simulink model "FullDPDDesign"  (R2015a)
settings: Solver=ode45  SolverMode=SingleTasking  StartTime=0.0  StopTime=1000000  RelTol=1e-3
undefined symbols (not defined in the file): CC1, CC2, gcbh, xlBlockLoadCallback, xlGetNormalizedPeriod, xlipgetpartsetting
libraries: xbsIndex_r4 x211
(part 2 of 2)

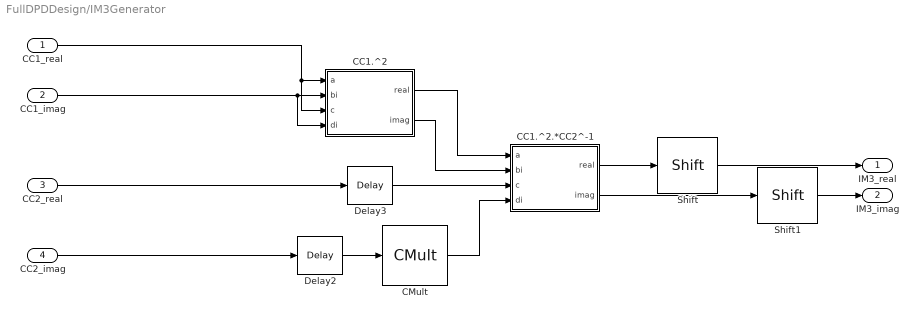
== system FullDPDDesign/IM3Generator ==
  CC1_real : Inport
  CC1_imag : Inport  Port=2
  CC2_real : Inport  Port=3
  CC2_imag : Inport  Port=4
  CC1.^2 : Subsystem
  CC1.^2.*CC2^-1 : Subsystem
  CMult : xbsIndex_r4/CMult  const=-1  gui_display_data_type=Fixed-point  const_n_bits=16  const_bin_pt=14  float_type=Single  exp_bits=8  fraction_bits=24  en=off  latency=0  precision=User Defined  arith_type="Signed  (2's comp)"  n_bits=16  bin_pt=14  quantization=Truncate  overflow=Wrap  dbl_ovrd=off  use_behavioral_HDL=off  mem_type=Distributed RAM  pipeline=off  block_type=cmult
  Delay2 : xbsIndex_r4/Delay  rst=off  infoeditControl=Selection of Reset will increase slice count due to use of real FFs and instead of SRLs  en=off  latency=4  dbl_ovrd=off  reg_retiming=off  block_type=delay
  Delay3 : xbsIndex_r4/Delay  rst=off  infoeditControl=Selection of Reset will increase slice count due to use of real FFs and instead of SRLs  en=off  latency=4  dbl_ovrd=off  reg_retiming=off  block_type=delay
  Shift : xbsIndex_r4/Shift  shift_dir=Left  shift_bits=2  en=off  latency=0  precision=Full  arith_type="Signed  (2's comp)"  n_bits=16  bin_pt=14  quantization=Truncate  overflow=Wrap  dbl_ovrd=off  block_type=shift
  Shift1 : xbsIndex_r4/Shift  shift_dir=Left  shift_bits=2  en=off  latency=0  precision=Full  arith_type="Signed  (2's comp)"  n_bits=16  bin_pt=14  quantization=Truncate  overflow=Wrap  dbl_ovrd=off  block_type=shift
  IM3_real : Outport
  IM3_imag : Outport  Port=2
  wires:
  CC1.^2/1(real) -> CC1.^2.*CC2^-1/1(a)
  Delay3/1 -> CC1.^2.*CC2^-1/3(c)
  CMult/1 -> CC1.^2.*CC2^-1/4(di)
  CC1.^2/2(imag) -> CC1.^2.*CC2^-1/2(bi)
  Delay2/1 -> CMult/1
  CC2_real/1 -> Delay3/1
  CC2_imag/1 -> Delay2/1
  CC1_real/1 -> CC1.^2/3(c), CC1.^2/1(a)
  CC1_imag/1 -> CC1.^2/2(bi), CC1.^2/4(di)
  CC1.^2.*CC2^-1/1(real) -> Shift/1
  CC1.^2.*CC2^-1/2(imag) -> Shift1/1
  Shift/1 -> IM3_real/1
  Shift1/1 -> IM3_imag/1

== system FullDPDDesign/IM3RotationGenerator ==
  Counter1 : xbsIndex_r4/Counter  cnt_type=Count Limited  cnt_to=39  operation=Up  start_count=0  cnt_by_val=1  arith_type=Unsigned  n_bits=6  bin_pt=0  load_pin=off  rst=off  en=off  explicit_period=on  period=1  dbl_ovrd=off  use_behavioral_HDL=off  implementation=Fabric  block_type=counter
  Negate1 : xbsIndex_r4/Negate  precision=User Defined  arith_type="Signed  (2's comp)"  n_bits=16  bin_pt=14  quantization=Truncate  overflow=Wrap  en=off  latency=0  dbl_ovrd=off  block_type=negate
  ROM : xbsIndex_r4/ROM  depth=40  initVector=cos(2*pi*(1:40)*9/40)  distributed_mem=Block RAM  rst=off  init_reg=0  en=off  latency=12  gui_display_data_type=Fixed-point  arith_type="Signed  (2's comp)"  n_bits=16  bin_pt=14  preci_type=Single  exp_width=8  frac_width=24  dbl_ovrd=off  optimize=Area  use_rpm=on  block_type=sprom
  ROM1 : xbsIndex_r4/ROM  depth=40  initVector=sin(2*pi*(1:40)*9/40)  distributed_mem=Block RAM  rst=off  init_reg=0  en=off  latency=12  gui_display_data_type=Fixed-point  arith_type="Signed  (2's comp)"  n_bits=16  bin_pt=14  preci_type=Single  exp_width=8  frac_width=24  dbl_ovrd=off  optimize=Area  use_rpm=on  block_type=sprom
  Rotate_real : Outport
  -Rotate_imag : Outport  Port=2
  Rotate_imag : Outport  Port=3
  wires:
  Counter1/1 -> ROM1/1, ROM/1
  ROM1/1 -> Negate1/1, Rotate_imag/1
  ROM/1 -> Rotate_real/1
  Negate1/1 -> -Rotate_imag/1

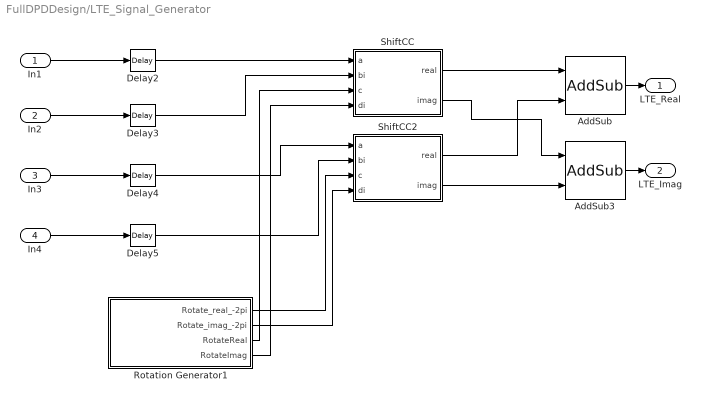
== system FullDPDDesign/LTE_Signal_Generator ==
  In1 : Inport
  In2 : Inport  Port=2
  In3 : Inport  Port=3
  In4 : Inport  Port=4
  AddSub : xbsIndex_r4/AddSub  mode=Addition  use_carryin=off  use_carryout=off  en=off  latency=3+8  precision=User Defined  arith_type="Signed  (2's comp)"  n_bits=16  bin_pt=14  quantization="Round  (unbiased: +/- Inf)"  overflow=Saturate  dbl_ovrd=off  use_behavioral_HDL=off  hw_selection=Fabric  pipelined=off  block_type=addsub
  AddSub3 : xbsIndex_r4/AddSub  mode=Addition  use_carryin=off  use_carryout=off  en=off  latency=3+8  precision=User Defined  arith_type="Signed  (2's comp)"  n_bits=16  bin_pt=14  quantization="Round  (unbiased: +/- Inf)"  overflow=Saturate  dbl_ovrd=off  use_behavioral_HDL=off  hw_selection=Fabric  pipelined=off  block_type=addsub
  Delay{2..5} (4 alike) : xbsIndex_r4/Delay  rst=off  infoeditControl=Selection of Reset will increase slice count due to use of real FFs and instead of SRLs  en=off  latency=1  dbl_ovrd=off  reg_retiming=off  block_type=delay
  Rotation Generator1 : Subsystem
  ShiftCC : Subsystem
  ShiftCC2 : Subsystem
  LTE_Real : Outport
  LTE_Imag : Outport  Port=2
  wires:
  In4/1 -> Delay5/1
  Delay3/1 -> ShiftCC/2(bi)
  Rotation Generator1/3(RotateReal) -> ShiftCC/3(c)
  Rotation Generator1/1(Rotate_real_-2pi) -> ShiftCC2/3(c)
  Delay5/1 -> ShiftCC2/2(bi)
  Delay4/1 -> ShiftCC2/1(a)
  Delay2/1 -> ShiftCC/1(a)
  Rotation Generator1/4(RotateImag) -> ShiftCC/4(di)
  In2/1 -> Delay3/1
  In3/1 -> Delay4/1
  Rotation Generator1/2(Rotate_imag_-2pi) -> ShiftCC2/4(di)
  ShiftCC/1(real) -> AddSub/1
  ShiftCC2/2(imag) -> AddSub3/2
  ShiftCC/2(imag) -> AddSub3/1
  ShiftCC2/1(real) -> AddSub/2
  AddSub3/1 -> LTE_Imag/1
  AddSub/1 -> LTE_Real/1
  In1/1 -> Delay2/1

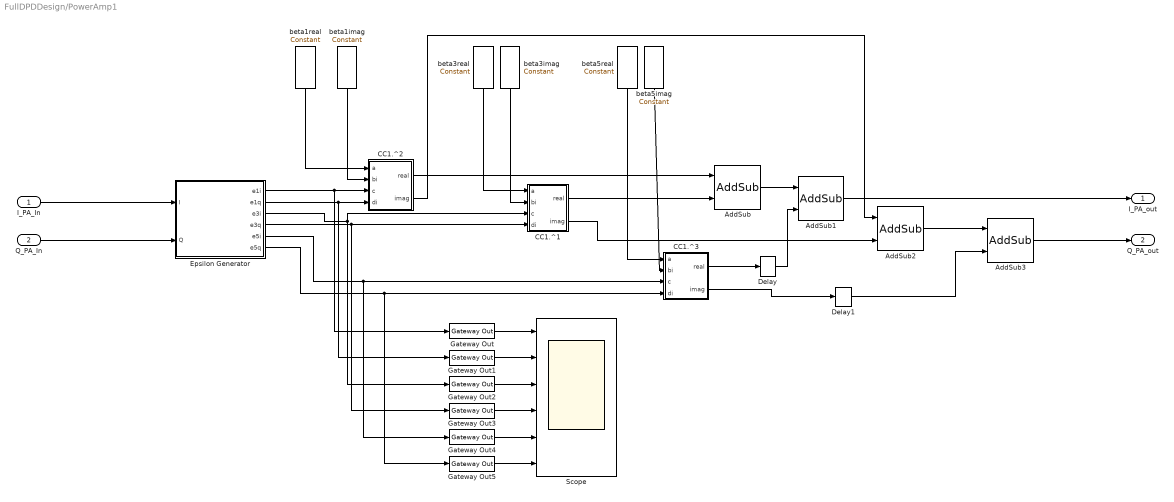
== system FullDPDDesign/PowerAmp1 ==
  I_PA_In : Inport
  Q_PA_In : Inport  Port=2
  AddSub{,1..3} (4 alike) : xbsIndex_r4/AddSub  mode=Addition  use_carryin=off  use_carryout=off  en=off  latency=1  precision=User Defined  arith_type="Signed  (2's comp)"  n_bits=32  bin_pt=28  quantization=Truncate  overflow=Saturate  dbl_ovrd=off  use_behavioral_HDL=off  hw_selection=Fabric  pipelined=off  block_type=addsub
  CC1.^1 : Subsystem
  CC1.^2 : Subsystem
  CC1.^3 : Subsystem
  Delay : xbsIndex_r4/Delay  rst=off  infoeditControl=Selection of Reset will increase slice count due to use of real FFs and instead of SRLs  en=off  latency=1  dbl_ovrd=off  reg_retiming=off  block_type=delay
  Delay1 : xbsIndex_r4/Delay  rst=off  infoeditControl=Selection of Reset will increase slice count due to use of real FFs and instead of SRLs  en=off  latency=1  dbl_ovrd=off  reg_retiming=off  block_type=delay
  Epsilon Generator : Subsystem
  Gateway Out{,1..5} (6 alike) : xbsIndex_r4/Gateway Out  inherit_from_input=off  hdl_port=on  timing_constraint=None  locs_specified=off  LOCs={}  UseAsDAC=off  DACChannel='1'  block_type=gatewayout
  Scope : Scope  NumInputPorts=6
      settings: YMin=-5~-5~-5~-5~-5~-5  YMax=5~5~5~5~5~5  SaveName=ScopeData3
  beta1imag : xbsIndex_r4/Constant  const=-0.0287  gui_display_data_type=Fixed-point  arith_type=Signed (2's comp)  n_bits=16  bin_pt=14  preci_type=Single  exp_width=8  frac_width=24  explicit_period=on  period=1  equ=P=C  opselect=C  inp2=PCIN>>17  opr=+  inp1=P  carry=CIN  dbl_ovrd=off  block_type=constant
  beta1real : xbsIndex_r4/Constant  const=1.0735  gui_display_data_type=Fixed-point  arith_type=Signed (2's comp)  n_bits=32  bin_pt=28  preci_type=Single  exp_width=8  frac_width=24  explicit_period=on  period=1  equ=P=C  opselect=C  inp2=PCIN>>17  opr=+  inp1=P  carry=CIN  dbl_ovrd=off  block_type=constant
  beta3imag : xbsIndex_r4/Constant  const=.1  gui_display_data_type=Fixed-point  arith_type=Signed (2's comp)  n_bits=32  bin_pt=28  preci_type=Single  exp_width=8  frac_width=24  explicit_period=on  period=1  equ=P=C  opselect=C  inp2=PCIN>>17  opr=+  inp1=P  carry=CIN  dbl_ovrd=off  block_type=constant
  beta3real : xbsIndex_r4/Constant  const=.2  gui_display_data_type=Fixed-point  arith_type=Signed (2's comp)  n_bits=32  bin_pt=28  preci_type=Single  exp_width=8  frac_width=24  explicit_period=on  period=1  equ=P=C  opselect=C  inp2=PCIN>>17  opr=+  inp1=P  carry=CIN  dbl_ovrd=off  block_type=constant
  beta5imag : xbsIndex_r4/Constant  const=0  gui_display_data_type=Fixed-point  arith_type=Signed (2's comp)  n_bits=32  bin_pt=28  preci_type=Single  exp_width=8  frac_width=24  explicit_period=on  period=1  equ=P=C  opselect=C  inp2=PCIN>>17  opr=+  inp1=P  carry=CIN  dbl_ovrd=off  block_type=constant
  beta5real : xbsIndex_r4/Constant  const=0  gui_display_data_type=Fixed-point  arith_type=Signed (2's comp)  n_bits=32  bin_pt=28  preci_type=Single  exp_width=8  frac_width=24  explicit_period=on  period=1  equ=P=C  opselect=C  inp2=PCIN>>17  opr=+  inp1=P  carry=CIN  dbl_ovrd=off  block_type=constant
  I_PA_out : Outport
  Q_PA_out : Outport  Port=2
  wires:
  I_PA_In/1 -> Epsilon Generator/1(I)
  CC1.^3/1(real) -> Delay/1
  CC1.^1/2(imag) -> AddSub2/2
  CC1.^1/1(real) -> AddSub/2
  CC1.^3/2(imag) -> Delay1/1
  Q_PA_In/1 -> Epsilon Generator/2(Q)
  CC1.^2/1(real) -> AddSub/1
  AddSub/1 -> AddSub1/1
  CC1.^2/2(imag) -> AddSub2/1
  AddSub2/1 -> AddSub3/1
  Epsilon Generator/1(e1i) -> CC1.^2/3(c), Gateway Out/1
  Epsilon Generator/2(e1q) -> CC1.^2/4(di), Gateway Out1/1
  beta1real/1 -> CC1.^2/1(a)
  beta1imag/1 -> CC1.^2/2(bi)
  Epsilon Generator/3(e3i) -> CC1.^1/3(c), Gateway Out2/1
  Epsilon Generator/4(e3q) -> CC1.^1/4(di), Gateway Out3/1
  beta3real/1 -> CC1.^1/1(a)
  beta3imag/1 -> CC1.^1/2(bi)
  beta5real/1 -> CC1.^3/1(a)
  beta5imag/1 -> CC1.^3/2(bi)
  Epsilon Generator/5(e5i) -> CC1.^3/3(c), Gateway Out4/1
  Epsilon Generator/6(e5q) -> CC1.^3/4(di), Gateway Out5/1
  Gateway Out/1 -> Scope/1
  Gateway Out1/1 -> Scope/2
  Gateway Out4/1 -> Scope/5
  Gateway Out5/1 -> Scope/6
  Gateway Out2/1 -> Scope/3
  Gateway Out3/1 -> Scope/4
  Delay/1 -> AddSub1/2
  Delay1/1 -> AddSub3/2
  AddSub1/1 -> I_PA_out/1
  AddSub3/1 -> Q_PA_out/1

== system FullDPDDesign/Predistorter ==
  DPD_real : Inport
  DPD_imag : Inport  Port=2
  LTE_real : Inport  Port=3
  LTE_imag : Inport  Port=4
  AddSub3 : xbsIndex_r4/AddSub  mode=Addition  use_carryin=off  use_carryout=off  en=off  latency=1  precision=User Defined  arith_type="Signed  (2's comp)"  n_bits=12  bin_pt=11  quantization=Truncate  overflow=Saturate  dbl_ovrd=off  use_behavioral_HDL=off  hw_selection=Fabric  pipelined=off  block_type=addsub
  AddSub4 : xbsIndex_r4/AddSub  mode=Addition  use_carryin=off  use_carryout=off  en=off  latency=1  precision=User Defined  arith_type="Signed  (2's comp)"  n_bits=12  bin_pt=11  quantization=Truncate  overflow=Saturate  dbl_ovrd=off  use_behavioral_HDL=off  hw_selection=Fabric  pipelined=off  block_type=addsub
  Out1 : Outport
  Out2 : Outport  Port=2
  wires:
  DPD_imag/1 -> AddSub3/1
  DPD_real/1 -> AddSub4/1
  LTE_imag/1 -> AddSub3/2
  AddSub3/1 -> Out2/1
  LTE_real/1 -> AddSub4/2
  AddSub4/1 -> Out1/1

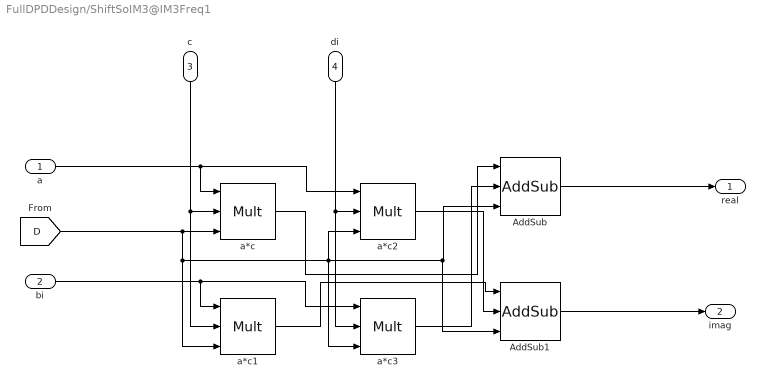
== system FullDPDDesign/ShiftSoIM3@IM3Freq1 ==
  a : Inport
  bi : Inport  Port=2
  c : Inport  Port=3
  di : Inport  Port=4
  AddSub : xbsIndex_r4/AddSub  mode=Subtraction  use_carryin=off  use_carryout=off  en=on  latency=1  precision=User Defined  arith_type="Signed  (2's comp)"  n_bits=16  bin_pt=14  quantization="Round  (unbiased: +/- Inf)"  overflow=Saturate  dbl_ovrd=off  use_behavioral_HDL=off  hw_selection=Fabric  pipelined=off  block_type=addsub
  AddSub1 : xbsIndex_r4/AddSub  mode=Addition  use_carryin=off  use_carryout=off  en=on  latency=1  precision=User Defined  arith_type="Signed  (2's comp)"  n_bits=16  bin_pt=14  quantization="Round  (unbiased: +/- Inf)"  overflow=Saturate  dbl_ovrd=off  use_behavioral_HDL=off  hw_selection=Fabric  pipelined=off  block_type=addsub
  a*c{,1..3} (4 alike) : xbsIndex_r4/Mult  precision=User Defined  arith_type="Signed  (2's comp)"  n_bits=16  bin_pt=14  quantization="Round  (unbiased: +/- Inf)"  overflow=Saturate  en=on  latency=3  dbl_ovrd=off  use_behavioral_HDL=off  opt=Speed  use_embedded=on  optimum_pipeline=off  pipeline=on  use_rpm=on  placement_style=Triangular  block_type=mult
  real : Outport
  imag : Outport  Port=2
  wires:
  a*c3/1 -> AddSub/2
  a*c1/1 -> AddSub1/1
  AddSub1/1 -> imag/1
  bi/1 -> a*c3/1, a*c1/1
  c/1 -> a*c1/2, a*c/2
  AddSub/1 -> real/1
  a*c/1 -> AddSub/1
  di/1 -> a*c3/2, a*c2/2
  a*c2/1 -> AddSub1/2
  a/1 -> a*c/1, a*c2/1
  [D] -> AddSub1/3, AddSub/3, a*c3/3, a*c2/3, a*c1/3, a*c/3

== system FullDPDDesign/ShiftSoIM3@IM3Freq2 ==
  a : Inport
  bi : Inport  Port=2
  c : Inport  Port=3
  di : Inport  Port=4
  AddSub : xbsIndex_r4/AddSub  mode=Subtraction  use_carryin=off  use_carryout=off  en=off  latency=1  precision=User Defined  arith_type="Signed  (2's comp)"  n_bits=16  bin_pt=14  quantization="Round  (unbiased: +/- Inf)"  overflow=Saturate  dbl_ovrd=off  use_behavioral_HDL=off  hw_selection=Fabric  pipelined=off  block_type=addsub
  AddSub1 : xbsIndex_r4/AddSub  mode=Addition  use_carryin=off  use_carryout=off  en=off  latency=1  precision=User Defined  arith_type="Signed  (2's comp)"  n_bits=16  bin_pt=14  quantization="Round  (unbiased: +/- Inf)"  overflow=Saturate  dbl_ovrd=off  use_behavioral_HDL=off  hw_selection=Fabric  pipelined=off  block_type=addsub
  a*c{,1..3} (4 alike) : xbsIndex_r4/Mult  precision=User Defined  arith_type="Signed  (2's comp)"  n_bits=16  bin_pt=14  quantization="Round  (unbiased: +/- Inf)"  overflow=Saturate  en=off  latency=3  dbl_ovrd=off  use_behavioral_HDL=off  opt=Speed  use_embedded=on  optimum_pipeline=off  pipeline=on  use_rpm=on  placement_style=Triangular  block_type=mult
  real : Outport
  imag : Outport  Port=2
  wires:
  a*c3/1 -> AddSub/2
  a*c1/1 -> AddSub1/1
  AddSub1/1 -> imag/1
  bi/1 -> a*c3/1, a*c1/1
  c/1 -> a*c/2, a*c1/2
  AddSub/1 -> real/1
  a*c/1 -> AddSub/1
  di/1 -> a*c2/2, a*c3/2
  a*c2/1 -> AddSub1/2
  a/1 -> a*c/1, a*c2/1

== system FullDPDDesign/Stream ==
  From Workspace10 : FromWorkspace  VariableName=CC2_real  SampleTime=0
  From Workspace11 : FromWorkspace  VariableName=CC2_imag  SampleTime=0
  From Workspace8 : FromWorkspace  VariableName=CC1_real  SampleTime=0
  From Workspace9 : FromWorkspace  VariableName=CC1_imag  SampleTime=0
  Gateway In{4..7} (4 alike) : xbsIndex_r4/Gateway In  gui_display_data_type=Fixed-point  arith_type="Signed  (2's comp)"  n_bits=16  bin_pt=14  preci_type=Single  exp_width=8  frac_width=24  quantization="Round  (unbiased: +/- Inf)"  overflow=Saturate  period=1  dbl_ovrd=off  timing_constraint=None  locs_specified=off  LOCs={}  UseAsADC=off  ADCChannel='1'  inherit_from_input=off  hdl_port=on  block_type=gatewayin
  Out1 : Outport
  Out2 : Outport  Port=2
  Out3 : Outport  Port=3
  Out4 : Outport  Port=4
  wires:
  From Workspace11/1 -> Gateway In7/1
  From Workspace10/1 -> Gateway In6/1
  From Workspace9/1 -> Gateway In5/1
  From Workspace8/1 -> Gateway In4/1
  Gateway In6/1 -> Out3/1
  Gateway In5/1 -> Out2/1
  Gateway In7/1 -> Out4/1
  Gateway In4/1 -> Out1/1

== system FullDPDDesign/Warp_PA ==
  In_I : Inport
  In_Q : Inport  Port=2
  FROM_PA_I : xbsIndex_r4/Gateway In  gui_display_data_type=Fixed-point  arith_type="Signed  (2's comp)"  n_bits=12  bin_pt=11  preci_type=Single  exp_width=8  frac_width=24  quantization="Round  (unbiased: +/- Inf)"  overflow=Saturate  period=1  dbl_ovrd=off  timing_constraint=None  locs_specified=off  LOCs={}  UseAsADC=off  ADCChannel='1'  inherit_from_input=off  hdl_port=on  block_type=gatewayin
  FROM_PA_Q : xbsIndex_r4/Gateway In  gui_display_data_type=Fixed-point  arith_type="Signed  (2's comp)"  n_bits=12  bin_pt=11  preci_type=Single  exp_width=8  frac_width=24  quantization="Round  (unbiased: +/- Inf)"  overflow=Saturate  period=1  dbl_ovrd=off  timing_constraint=None  locs_specified=off  LOCs={}  UseAsADC=off  ADCChannel='1'  inherit_from_input=off  hdl_port=on  block_type=gatewayin
  TO_PA_I : xbsIndex_r4/Gateway Out  inherit_from_input=off  hdl_port=on  timing_constraint=None  locs_specified=off  LOCs={}  UseAsDAC=off  DACChannel='1'  block_type=gatewayout
  TO_PA_Q : xbsIndex_r4/Gateway Out  inherit_from_input=off  hdl_port=on  timing_constraint=None  locs_specified=off  LOCs={}  UseAsDAC=off  DACChannel='1'  block_type=gatewayout
  Out_I : Outport
  Out_Q : Outport  Port=2
  wires:
  In_Q/1 -> TO_PA_Q/1
  FROM_PA_I/1 -> Out_I/1
  In_I/1 -> TO_PA_I/1
  FROM_PA_Q/1 -> Out_Q/1

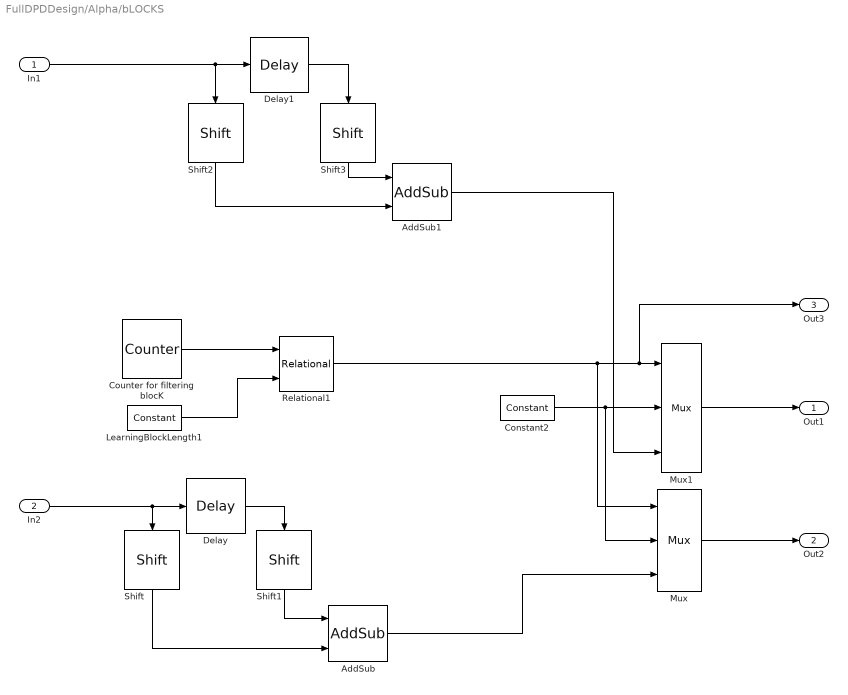
== system FullDPDDesign/Alpha/bLOCKS ==
  In1 : Inport
  In2 : Inport  Port=2
  AddSub : xbsIndex_r4/AddSub  mode=Addition  use_carryin=off  use_carryout=off  en=off  latency=1  precision=User Defined  arith_type="Signed  (2's comp)"  n_bits=16  bin_pt=14  quantization=Truncate  overflow=Saturate  dbl_ovrd=off  use_behavioral_HDL=off  hw_selection=Fabric  pipelined=off  block_type=addsub
  AddSub1 : xbsIndex_r4/AddSub  mode=Addition  use_carryin=off  use_carryout=off  en=off  latency=1  precision=User Defined  arith_type="Signed  (2's comp)"  n_bits=16  bin_pt=14  quantization=Truncate  overflow=Saturate  dbl_ovrd=off  use_behavioral_HDL=off  hw_selection=Fabric  pipelined=off  block_type=addsub
  Constant2 : xbsIndex_r4/Constant  const=0  gui_display_data_type=Fixed-point  arith_type=Signed (2's comp)  n_bits=16  bin_pt=14  preci_type=Single  exp_width=8  frac_width=24  explicit_period=on  period=1  equ=P=C  opselect=C  inp2=PCIN>>17  opr=+  inp1=P  carry=CIN  dbl_ovrd=off  block_type=constant
  Counter for filtering blocK : xbsIndex_r4/Counter  cnt_type=Free Running  cnt_to=2^9-1  operation=Up  start_count=0  cnt_by_val=1  arith_type=Unsigned  n_bits=8  bin_pt=0  load_pin=off  rst=off  en=off  explicit_period=on  period=1  dbl_ovrd=off  use_behavioral_HDL=off  implementation=Fabric  block_type=counter
  Delay : xbsIndex_r4/Delay  rst=off  infoeditControl=Selection of Reset will increase slice count due to use of real FFs and instead of SRLs  en=off  latency=1  dbl_ovrd=off  reg_retiming=off  block_type=delay
  Delay1 : xbsIndex_r4/Delay  rst=off  infoeditControl=Selection of Reset will increase slice count due to use of real FFs and instead of SRLs  en=off  latency=1  dbl_ovrd=off  reg_retiming=off  block_type=delay
  LearningBlockLength1 : xbsIndex_r4/Constant  const=0  gui_display_data_type=Fixed-point  arith_type=Unsigned  n_bits=1  bin_pt=0  preci_type=Single  exp_width=8  frac_width=24  explicit_period=off  period=1  equ=P=C  opselect=C  inp2=PCIN>>17  opr=+  inp1=P  carry=CIN  dbl_ovrd=off  block_type=constant
  Mux : xbsIndex_r4/Mux  inputs=2  en=off  latency=0  precision=User Defined  arith_type="Signed  (2's comp)"  n_bits=16  bin_pt=14  quantization=Truncate  overflow=Saturate  dbl_ovrd=off  block_type=mux
  Mux1 : xbsIndex_r4/Mux  inputs=2  en=off  latency=0  precision=User Defined  arith_type="Signed  (2's comp)"  n_bits=16  bin_pt=14  quantization=Truncate  overflow=Saturate  dbl_ovrd=off  block_type=mux
  Relational1 : xbsIndex_r4/Relational  mode=a=b  en=off  latency=0  dbl_ovrd=off  block_type=relational
  Shift{,1..3} (4 alike) : xbsIndex_r4/Shift  shift_dir=Right  shift_bits=1  en=off  latency=0  precision=Full  arith_type="Signed  (2's comp)"  n_bits=16  bin_pt=14  quantization=Truncate  overflow=Wrap  dbl_ovrd=off  block_type=shift
  Out1 : Outport
  Out2 : Outport  Port=2
  Out3 : Outport  Port=3
  wires:
  Counter for filtering blocK/1 -> Relational1/1
  Constant2/1 -> Mux/2, Mux1/2
  Mux1/1 -> Out1/1
  LearningBlockLength1/1 -> Relational1/2
  AddSub1/1 -> Mux1/3
  In2/1 -> Shift/1, Delay/1
  Mux/1 -> Out2/1
  Delay/1 -> Shift1/1
  Shift1/1 -> AddSub/1
  Shift/1 -> AddSub/2
  AddSub/1 -> Mux/3
  In1/1 -> Shift2/1, Delay1/1
  Delay1/1 -> Shift3/1
  Shift3/1 -> AddSub1/1
  Shift2/1 -> AddSub1/2
  Relational1/1 -> Out3/1, Mux1/1, Mux/1

== system FullDPDDesign/IM3Generator/CC1.^2 ==
  a : Inport
  bi : Inport  Port=2
  c : Inport  Port=3
  di : Inport  Port=4
  AddSub : xbsIndex_r4/AddSub  mode=Subtraction  use_carryin=off  use_carryout=off  en=off  latency=1  precision=User Defined  arith_type="Signed  (2's comp)"  n_bits=16  bin_pt=14  quantization="Round  (unbiased: +/- Inf)"  overflow=Saturate  dbl_ovrd=off  use_behavioral_HDL=off  hw_selection=Fabric  pipelined=off  block_type=addsub
  AddSub1 : xbsIndex_r4/AddSub  mode=Addition  use_carryin=off  use_carryout=off  en=off  latency=1  precision=User Defined  arith_type="Signed  (2's comp)"  n_bits=16  bin_pt=14  quantization="Round  (unbiased: +/- Inf)"  overflow=Saturate  dbl_ovrd=off  use_behavioral_HDL=off  hw_selection=Fabric  pipelined=off  block_type=addsub
  a*c{,1..3} (4 alike) : xbsIndex_r4/Mult  precision=User Defined  arith_type="Signed  (2's comp)"  n_bits=16  bin_pt=14  quantization="Round  (unbiased: +/- Inf)"  overflow=Saturate  en=off  latency=3  dbl_ovrd=off  use_behavioral_HDL=off  opt=Speed  use_embedded=on  optimum_pipeline=off  pipeline=on  use_rpm=on  placement_style=Triangular  block_type=mult
  real : Outport
  imag : Outport  Port=2
  wires:
  a*c3/1 -> AddSub/2
  a*c1/1 -> AddSub1/1
  AddSub1/1 -> imag/1
  bi/1 -> a*c3/1, a*c1/1
  c/1 -> a*c/2, a*c1/2
  AddSub/1 -> real/1
  a*c/1 -> AddSub/1
  di/1 -> a*c2/2, a*c3/2
  a*c2/1 -> AddSub1/2
  a/1 -> a*c/1, a*c2/1

== system FullDPDDesign/IM3Generator/CC1.^2.*CC2^-1 ==
  a : Inport
  bi : Inport  Port=2
  c : Inport  Port=3
  di : Inport  Port=4
  AddSub : xbsIndex_r4/AddSub  mode=Subtraction  use_carryin=off  use_carryout=off  en=off  latency=1  precision=User Defined  arith_type="Signed  (2's comp)"  n_bits=16  bin_pt=14  quantization="Round  (unbiased: +/- Inf)"  overflow=Saturate  dbl_ovrd=off  use_behavioral_HDL=off  hw_selection=Fabric  pipelined=off  block_type=addsub
  AddSub1 : xbsIndex_r4/AddSub  mode=Addition  use_carryin=off  use_carryout=off  en=off  latency=1  precision=User Defined  arith_type="Signed  (2's comp)"  n_bits=16  bin_pt=14  quantization="Round  (unbiased: +/- Inf)"  overflow=Saturate  dbl_ovrd=off  use_behavioral_HDL=off  hw_selection=Fabric  pipelined=off  block_type=addsub
  a*c{,1..3} (4 alike) : xbsIndex_r4/Mult  precision=User Defined  arith_type="Signed  (2's comp)"  n_bits=16  bin_pt=14  quantization="Round  (unbiased: +/- Inf)"  overflow=Saturate  en=off  latency=3  dbl_ovrd=off  use_behavioral_HDL=off  opt=Speed  use_embedded=on  optimum_pipeline=off  pipeline=on  use_rpm=on  placement_style=Triangular  block_type=mult
  real : Outport
  imag : Outport  Port=2
  wires:
  a*c3/1 -> AddSub/2
  a*c1/1 -> AddSub1/1
  AddSub1/1 -> imag/1
  bi/1 -> a*c3/1, a*c1/1
  c/1 -> a*c/2, a*c1/2
  AddSub/1 -> real/1
  a*c/1 -> AddSub/1
  di/1 -> a*c2/2, a*c3/2
  a*c2/1 -> AddSub1/2
  a/1 -> a*c/1, a*c2/1

== system FullDPDDesign/LTE_Signal_Generator/Rotation Generator1 ==
  Counter1 : xbsIndex_r4/Counter  cnt_type=Count Limited  cnt_to=39  operation=Up  start_count=0  cnt_by_val=1  arith_type=Unsigned  n_bits=6  bin_pt=0  load_pin=off  rst=off  en=off  explicit_period=on  period=1  dbl_ovrd=off  use_behavioral_HDL=off  implementation=Fabric  block_type=counter
  Negate1 : xbsIndex_r4/Negate  precision=User Defined  arith_type="Signed  (2's comp)"  n_bits=16  bin_pt=14  quantization=Truncate  overflow=Wrap  en=off  latency=0  dbl_ovrd=off  block_type=negate
  ROM : xbsIndex_r4/ROM  depth=40  initVector=cos(2*pi*(1:40)*3/40)  distributed_mem=Block RAM  rst=off  init_reg=0  en=off  latency=1  gui_display_data_type=Fixed-point  arith_type="Signed  (2's comp)"  n_bits=16  bin_pt=14  preci_type=Single  exp_width=8  frac_width=24  dbl_ovrd=off  optimize=Area  use_rpm=on  block_type=sprom
  ROM1 : xbsIndex_r4/ROM  depth=40  initVector=sin(2*pi*(1:40)*3/40)  distributed_mem=Block RAM  rst=off  init_reg=0  en=off  latency=1  gui_display_data_type=Fixed-point  arith_type="Signed  (2's comp)"  n_bits=16  bin_pt=14  preci_type=Single  exp_width=8  frac_width=24  dbl_ovrd=off  optimize=Area  use_rpm=on  block_type=sprom
  Rotate_real_-2pi : Outport
  Rotate_imag_-2pi : Outport  Port=2
  RotateReal : Outport  Port=3
  RotateImag : Outport  Port=4
  wires:
  Counter1/1 -> ROM1/1, ROM/1
  ROM1/1 -> Negate1/1, RotateImag/1
  ROM/1 -> RotateReal/1, Rotate_real_-2pi/1
  Negate1/1 -> Rotate_imag_-2pi/1

== system FullDPDDesign/LTE_Signal_Generator/ShiftCC ==
  a : Inport
  bi : Inport  Port=2
  c : Inport  Port=3
  di : Inport  Port=4
  AddSub : xbsIndex_r4/AddSub  mode=Subtraction  use_carryin=off  use_carryout=off  en=off  latency=1  precision=User Defined  arith_type="Signed  (2's comp)"  n_bits=16  bin_pt=14  quantization="Round  (unbiased: +/- Inf)"  overflow=Saturate  dbl_ovrd=off  use_behavioral_HDL=off  hw_selection=Fabric  pipelined=off  block_type=addsub
  AddSub1 : xbsIndex_r4/AddSub  mode=Addition  use_carryin=off  use_carryout=off  en=off  latency=1  precision=User Defined  arith_type="Signed  (2's comp)"  n_bits=16  bin_pt=14  quantization="Round  (unbiased: +/- Inf)"  overflow=Saturate  dbl_ovrd=off  use_behavioral_HDL=off  hw_selection=Fabric  pipelined=off  block_type=addsub
  a*c{,1..3} (4 alike) : xbsIndex_r4/Mult  precision=User Defined  arith_type="Signed  (2's comp)"  n_bits=16  bin_pt=14  quantization="Round  (unbiased: +/- Inf)"  overflow=Saturate  en=off  latency=3  dbl_ovrd=off  use_behavioral_HDL=off  opt=Speed  use_embedded=on  optimum_pipeline=off  pipeline=on  use_rpm=on  placement_style=Triangular  block_type=mult
  real : Outport
  imag : Outport  Port=2
  wires:
  a*c3/1 -> AddSub/2
  a*c1/1 -> AddSub1/1
  AddSub1/1 -> imag/1
  bi/1 -> a*c3/1, a*c1/1
  c/1 -> a*c/2, a*c1/2
  AddSub/1 -> real/1
  a*c/1 -> AddSub/1
  di/1 -> a*c2/2, a*c3/2
  a*c2/1 -> AddSub1/2
  a/1 -> a*c/1, a*c2/1

== system FullDPDDesign/LTE_Signal_Generator/ShiftCC2 ==
  a : Inport
  bi : Inport  Port=2
  c : Inport  Port=3
  di : Inport  Port=4
  AddSub : xbsIndex_r4/AddSub  mode=Subtraction  use_carryin=off  use_carryout=off  en=off  latency=1  precision=User Defined  arith_type="Signed  (2's comp)"  n_bits=16  bin_pt=14  quantization="Round  (unbiased: +/- Inf)"  overflow=Saturate  dbl_ovrd=off  use_behavioral_HDL=off  hw_selection=Fabric  pipelined=off  block_type=addsub
  AddSub1 : xbsIndex_r4/AddSub  mode=Addition  use_carryin=off  use_carryout=off  en=off  latency=1  precision=User Defined  arith_type="Signed  (2's comp)"  n_bits=16  bin_pt=14  quantization="Round  (unbiased: +/- Inf)"  overflow=Saturate  dbl_ovrd=off  use_behavioral_HDL=off  hw_selection=Fabric  pipelined=off  block_type=addsub
  a*c{,1..3} (4 alike) : xbsIndex_r4/Mult  precision=User Defined  arith_type="Signed  (2's comp)"  n_bits=16  bin_pt=14  quantization="Round  (unbiased: +/- Inf)"  overflow=Saturate  en=off  latency=3  dbl_ovrd=off  use_behavioral_HDL=off  opt=Speed  use_embedded=on  optimum_pipeline=off  pipeline=on  use_rpm=on  placement_style=Triangular  block_type=mult
  real : Outport
  imag : Outport  Port=2
  wires:
  a*c3/1 -> AddSub/2
  a*c1/1 -> AddSub1/1
  AddSub1/1 -> imag/1
  bi/1 -> a*c3/1, a*c1/1
  c/1 -> a*c/2, a*c1/2
  AddSub/1 -> real/1
  a*c/1 -> AddSub/1
  di/1 -> a*c2/2, a*c3/2
  a*c2/1 -> AddSub1/2
  a/1 -> a*c/1, a*c2/1

== system FullDPDDesign/PowerAmp1/CC1.^1 ==
  a : Inport
  bi : Inport  Port=2
  c : Inport  Port=3
  di : Inport  Port=4
  AddSub : xbsIndex_r4/AddSub  mode=Subtraction  use_carryin=off  use_carryout=off  en=off  latency=1  precision=User Defined  arith_type="Signed  (2's comp)"  n_bits=32  bin_pt=28  quantization="Round  (unbiased: +/- Inf)"  overflow=Saturate  dbl_ovrd=off  use_behavioral_HDL=off  hw_selection=Fabric  pipelined=off  block_type=addsub
  AddSub1 : xbsIndex_r4/AddSub  mode=Addition  use_carryin=off  use_carryout=off  en=off  latency=1  precision=User Defined  arith_type="Signed  (2's comp)"  n_bits=32  bin_pt=28  quantization="Round  (unbiased: +/- Inf)"  overflow=Saturate  dbl_ovrd=off  use_behavioral_HDL=off  hw_selection=Fabric  pipelined=off  block_type=addsub
  a*c{,1..3} (4 alike) : xbsIndex_r4/Mult  precision=User Defined  arith_type="Signed  (2's comp)"  n_bits=32  bin_pt=28  quantization="Round  (unbiased: +/- Inf)"  overflow=Saturate  en=off  latency=3  dbl_ovrd=off  use_behavioral_HDL=off  opt=Speed  use_embedded=on  optimum_pipeline=off  pipeline=on  use_rpm=on  placement_style=Triangular  block_type=mult
  real : Outport
  imag : Outport  Port=2
  wires:
  a*c2/1 -> AddSub/2
  a*c3/1 -> AddSub1/1
  AddSub1/1 -> imag/1
  bi/1 -> a*c2/1, a*c3/1
  c/1 -> a*c3/2, a*c/2
  AddSub/1 -> real/1
  a*c/1 -> AddSub/1
  di/1 -> a*c2/2, a*c1/2
  a*c1/1 -> AddSub1/2
  a/1 -> a*c1/1, a*c/1

== system FullDPDDesign/PowerAmp1/CC1.^2 ==
  a : Inport
  bi : Inport  Port=2
  c : Inport  Port=3
  di : Inport  Port=4
  AddSub : xbsIndex_r4/AddSub  mode=Subtraction  use_carryin=off  use_carryout=off  en=off  latency=1  precision=User Defined  arith_type="Signed  (2's comp)"  n_bits=32  bin_pt=28  quantization="Round  (unbiased: +/- Inf)"  overflow=Saturate  dbl_ovrd=off  use_behavioral_HDL=off  hw_selection=Fabric  pipelined=off  block_type=addsub
  AddSub1 : xbsIndex_r4/AddSub  mode=Addition  use_carryin=off  use_carryout=off  en=off  latency=1  precision=User Defined  arith_type="Signed  (2's comp)"  n_bits=32  bin_pt=28  quantization="Round  (unbiased: +/- Inf)"  overflow=Saturate  dbl_ovrd=off  use_behavioral_HDL=off  hw_selection=Fabric  pipelined=off  block_type=addsub
  a*c{,1..3} (4 alike) : xbsIndex_r4/Mult  precision=User Defined  arith_type="Signed  (2's comp)"  n_bits=32  bin_pt=28  quantization="Round  (unbiased: +/- Inf)"  overflow=Saturate  en=off  latency=3  dbl_ovrd=off  use_behavioral_HDL=off  opt=Speed  use_embedded=on  optimum_pipeline=off  pipeline=on  use_rpm=on  placement_style=Triangular  block_type=mult
  real : Outport
  imag : Outport  Port=2
  wires:
  a*c2/1 -> AddSub/2
  a*c3/1 -> AddSub1/1
  AddSub1/1 -> imag/1
  bi/1 -> a*c2/1, a*c3/1
  c/1 -> a*c3/2, a*c/2
  AddSub/1 -> real/1
  a*c/1 -> AddSub/1
  di/1 -> a*c2/2, a*c1/2
  a*c1/1 -> AddSub1/2
  a/1 -> a*c1/1, a*c/1

== system FullDPDDesign/PowerAmp1/CC1.^3 ==
  a : Inport
  bi : Inport  Port=2
  c : Inport  Port=3
  di : Inport  Port=4
  AddSub : xbsIndex_r4/AddSub  mode=Subtraction  use_carryin=off  use_carryout=off  en=off  latency=1  precision=User Defined  arith_type="Signed  (2's comp)"  n_bits=32  bin_pt=28  quantization="Round  (unbiased: +/- Inf)"  overflow=Saturate  dbl_ovrd=off  use_behavioral_HDL=off  hw_selection=Fabric  pipelined=off  block_type=addsub
  AddSub1 : xbsIndex_r4/AddSub  mode=Addition  use_carryin=off  use_carryout=off  en=off  latency=1  precision=User Defined  arith_type="Signed  (2's comp)"  n_bits=32  bin_pt=28  quantization="Round  (unbiased: +/- Inf)"  overflow=Saturate  dbl_ovrd=off  use_behavioral_HDL=off  hw_selection=Fabric  pipelined=off  block_type=addsub
  a*c{,1..3} (4 alike) : xbsIndex_r4/Mult  precision=User Defined  arith_type="Signed  (2's comp)"  n_bits=32  bin_pt=28  quantization="Round  (unbiased: +/- Inf)"  overflow=Saturate  en=off  latency=3  dbl_ovrd=off  use_behavioral_HDL=off  opt=Speed  use_embedded=on  optimum_pipeline=off  pipeline=on  use_rpm=on  placement_style=Triangular  block_type=mult
  real : Outport
  imag : Outport  Port=2
  wires:
  a*c2/1 -> AddSub/2
  a*c3/1 -> AddSub1/1
  AddSub1/1 -> imag/1
  bi/1 -> a*c2/1, a*c3/1
  c/1 -> a*c3/2, a*c/2
  AddSub/1 -> real/1
  a*c/1 -> AddSub/1
  di/1 -> a*c2/2, a*c1/2
  a*c1/1 -> AddSub1/2
  a/1 -> a*c1/1, a*c/1

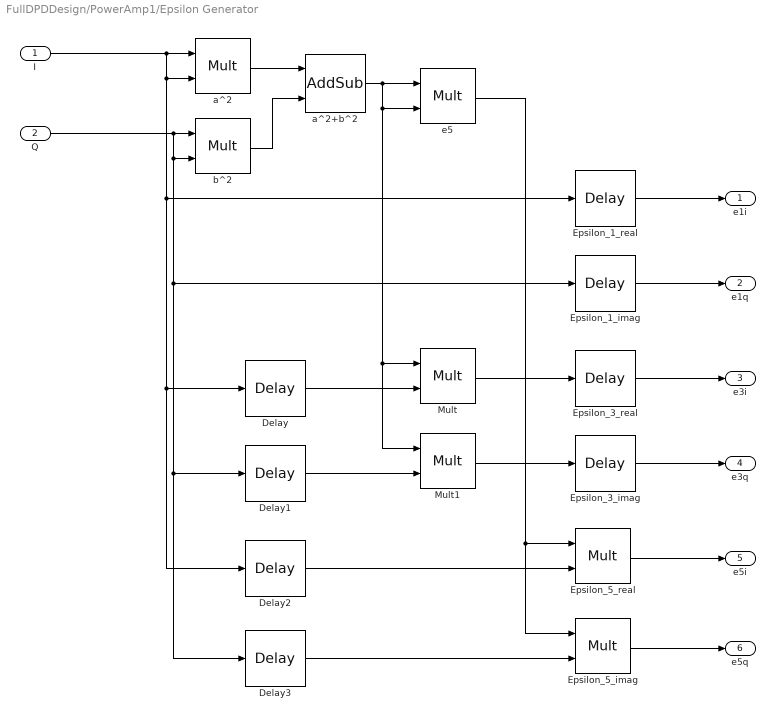
== system FullDPDDesign/PowerAmp1/Epsilon Generator ==
  I : Inport
  Q : Inport  Port=2
  Delay : xbsIndex_r4/Delay  rst=off  infoeditControl=Selection of Reset will increase slice count due to use of real FFs and instead of SRLs  en=off  latency=4  dbl_ovrd=off  reg_retiming=off  block_type=delay
  Delay1 : xbsIndex_r4/Delay  rst=off  infoeditControl=Selection of Reset will increase slice count due to use of real FFs and instead of SRLs  en=off  latency=4  dbl_ovrd=off  reg_retiming=off  block_type=delay
  Delay2 : xbsIndex_r4/Delay  rst=off  infoeditControl=Selection of Reset will increase slice count due to use of real FFs and instead of SRLs  en=off  latency=7  dbl_ovrd=off  reg_retiming=off  block_type=delay
  Delay3 : xbsIndex_r4/Delay  rst=off  infoeditControl=Selection of Reset will increase slice count due to use of real FFs and instead of SRLs  en=off  latency=7  dbl_ovrd=off  reg_retiming=off  block_type=delay
  Epsilon_1_imag : xbsIndex_r4/Delay  rst=off  infoeditControl=Selection of Reset will increase slice count due to use of real FFs and instead of SRLs  en=off  latency=10  dbl_ovrd=off  reg_retiming=off  block_type=delay
  Epsilon_1_real : xbsIndex_r4/Delay  rst=off  infoeditControl=Selection of Reset will increase slice count due to use of real FFs and instead of SRLs  en=off  latency=10  dbl_ovrd=off  reg_retiming=off  block_type=delay
  Epsilon_3_imag : xbsIndex_r4/Delay  rst=off  infoeditControl=Selection of Reset will increase slice count due to use of real FFs and instead of SRLs  en=off  latency=3  dbl_ovrd=off  reg_retiming=off  block_type=delay
  Epsilon_3_real : xbsIndex_r4/Delay  rst=off  infoeditControl=Selection of Reset will increase slice count due to use of real FFs and instead of SRLs  en=off  latency=3  dbl_ovrd=off  reg_retiming=off  block_type=delay
  Epsilon_5_imag : xbsIndex_r4/Mult  precision=User Defined  arith_type="Signed  (2's comp)"  n_bits=32  bin_pt=28  quantization=Truncate  overflow=Saturate  en=off  latency=3  dbl_ovrd=off  use_behavioral_HDL=off  opt=Speed  use_embedded=on  optimum_pipeline=off  pipeline=on  use_rpm=on  placement_style=Triangular  block_type=mult
  Epsilon_5_real : xbsIndex_r4/Mult  precision=User Defined  arith_type="Signed  (2's comp)"  n_bits=32  bin_pt=28  quantization=Truncate  overflow=Saturate  en=off  latency=3  dbl_ovrd=off  use_behavioral_HDL=off  opt=Speed  use_embedded=on  optimum_pipeline=off  pipeline=on  use_rpm=on  placement_style=Triangular  block_type=mult
  Mult : xbsIndex_r4/Mult  precision=User Defined  arith_type="Signed  (2's comp)"  n_bits=32  bin_pt=28  quantization=Truncate  overflow=Saturate  en=off  latency=3  dbl_ovrd=off  use_behavioral_HDL=off  opt=Speed  use_embedded=on  optimum_pipeline=off  pipeline=on  use_rpm=on  placement_style=Triangular  block_type=mult
  Mult1 : xbsIndex_r4/Mult  precision=User Defined  arith_type="Signed  (2's comp)"  n_bits=32  bin_pt=28  quantization=Truncate  overflow=Saturate  en=off  latency=3  dbl_ovrd=off  use_behavioral_HDL=off  opt=Speed  use_embedded=on  optimum_pipeline=off  pipeline=on  use_rpm=on  placement_style=Triangular  block_type=mult
  a^2 : xbsIndex_r4/Mult  precision=User Defined  arith_type="Signed  (2's comp)"  n_bits=32  bin_pt=28  quantization=Truncate  overflow=Saturate  en=off  latency=3  dbl_ovrd=off  use_behavioral_HDL=off  opt=Speed  use_embedded=on  optimum_pipeline=off  pipeline=on  use_rpm=on  placement_style=Triangular  block_type=mult
  a^2+b^2 : xbsIndex_r4/AddSub  mode=Addition  use_carryin=off  use_carryout=off  en=off  latency=1  precision=User Defined  arith_type="Signed  (2's comp)"  n_bits=32  bin_pt=28  quantization=Truncate  overflow=Saturate  dbl_ovrd=off  use_behavioral_HDL=off  hw_selection=Fabric  pipelined=off  block_type=addsub
  b^2 : xbsIndex_r4/Mult  precision=User Defined  arith_type="Signed  (2's comp)"  n_bits=32  bin_pt=28  quantization=Truncate  overflow=Saturate  en=off  latency=3  dbl_ovrd=off  use_behavioral_HDL=off  opt=Speed  use_embedded=on  optimum_pipeline=off  pipeline=on  use_rpm=on  placement_style=Triangular  block_type=mult
  e5 : xbsIndex_r4/Mult  precision=User Defined  arith_type="Signed  (2's comp)"  n_bits=32  bin_pt=28  quantization=Truncate  overflow=Saturate  en=off  latency=3  dbl_ovrd=off  use_behavioral_HDL=off  opt=Speed  use_embedded=on  optimum_pipeline=off  pipeline=on  use_rpm=on  placement_style=Triangular  block_type=mult
  e1i : Outport
  e1q : Outport  Port=2
  e3i : Outport  Port=3
  e3q : Outport  Port=4
  e5i : Outport  Port=5
  e5q : Outport  Port=6
  wires:
  a^2+b^2/1 -> Mult1/1, Mult/1, e5/2, e5/1
  a^2/1 -> a^2+b^2/1
  I/1 -> Epsilon_1_real/1, Delay2/1, Delay/1, a^2/2, a^2/1
  b^2/1 -> a^2+b^2/2
  Q/1 -> Delay3/1, Delay1/1, Epsilon_1_imag/1, b^2/2, b^2/1
  Delay/1 -> Mult/2
  Delay1/1 -> Mult1/2
  e5/1 -> Epsilon_5_imag/1, Epsilon_5_real/1
  Delay2/1 -> Epsilon_5_real/2
  Delay3/1 -> Epsilon_5_imag/2
  Mult/1 -> Epsilon_3_real/1
  Mult1/1 -> Epsilon_3_imag/1
  Epsilon_1_real/1 -> e1i/1
  Epsilon_1_imag/1 -> e1q/1
  Epsilon_3_real/1 -> e3i/1
  Epsilon_3_imag/1 -> e3q/1
  Epsilon_5_real/1 -> e5i/1
  Epsilon_5_imag/1 -> e5q/1
